simulink model "First_HIL_Scenario2"  (R2023a)
settings: Solver=ode1  StartTime=0.0  StopTime=inf  FixedStep=0.001  RelTol=1e-3
undefined symbols (not defined in the file or in its folder): ACC_X, ACC_Y, ACC_Z, Altitude, distance, GetTimeDemo, Gyro_X, Gyro_Y, Gyro_Z, Heading, Lane_Car_Distance_Left, Lane_Car_Distance_Right, Lane_Class, Lane_Coefficient_C0, Lane_Coefficient_C1, Lane_Coefficient_C2, Lane_Coefficient_C3, Lane_Curvature, Lane_Distance, Lane_ID, Latitude, Longitude, OBJ_Class, OBJ_Height, OBJ_ID, OBJ_Length, OBJ_RCS, OBJ_S_Azimuth, OBJ_S_Elevation, OBJ_S_Range, OBJ_S_Velocity, OBJ_Velocity, OBJ_Width, OBJ_X, OBJ_Y, OBJ_Z, Pitch, Roll, Subsystem, time, Timestamp, TrafficLight_Direction, TrafficLight_State, TrafficLight_Timer, Velocity, width, x, x1, x2, x3, x4, y, y1, y2, y3, y4, Yaw
(part 1 of 4)
Description:
  | 22222
settings Model: Creator=15751  LastModifiedBy=owner
settings SolverCC: AlgebraicLoopSolver=TrustRegion
settings OptimizationCC: LifeSpan=inf
settings DebuggingCC: MultiTaskRateTransMsg=warning  UnconnectedInputMsg=warning  UnconnectedOutputMsg=warning  UnconnectedLineMsg=warning  RootOutportRequireBusObject=error  StrictBusMsg=ErrorOnBusTreatedAsVector  ArithmeticOperatorsInVariantConditions=warning
settings HardwareCC: ProdBitPerPointer=32  ProdBitPerSizeT=32  ProdBitPerPtrDiffT=32  ProdLargestAtomicFloat=None  ProdWordSize=32  ProdHWDeviceType=Intel->x86/Pentium
settings ModelReferenceCC: EnableRefExpFcnMdlSchedulingChecks=on
settings SFSimCC: CustomCodeUndefinedFunction=UseInterfaceOnly
settings RTWCC: Description=NI Phar Lap Real-Time & Windows Targets  SystemTargetFile=NIVeriStand.tlc  TemplateMakefile=NIVeriStand_vc.tmf
settings RTWCC: CustomInclude=|
  | C:\Program Files\PanoSim5\Bin\SimulinkLib\dependence\NI
  | C:\Program
  | Files\PanoSim5\Bin\SimulinkLib\dependence\NI
settings RTWCC: CustomSource=|
  | DataReceiver.c
  | DataSender.c
  | udpFunc.c
settings CodeAppCC: StateflowObjectComments=on
settings STFCustomTargetCC: TargetLangStandard=C89/C90 (ANSI)  ConcurrentExecutionCompliant=off  MatFileLogging=on  MATLABClassNameForMDSCustomization=Simulink.SoftwareTarget.TargetSpecificTriggerConfigurationBase  UseToolchainInfoCompliant=off  SystemTargetFile=NIVeriStand.tlc
settings SimscapeCC: SimscapeNormalizeSystem=off

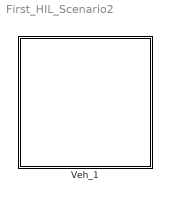
== system First_HIL_Scenario2 ==
  Veh_1 : Subsystem  Tag=PanoSim_System
      mask Display: image(imread('Sedan_2.jpg'));color('white');text(0,0,'Veh_1','HorizontalAlignment','left','verticalAlignment','bottom');color('red');text(0.1,0.1,'P','HorizontalAlignment','right','verticalAlignment','top');

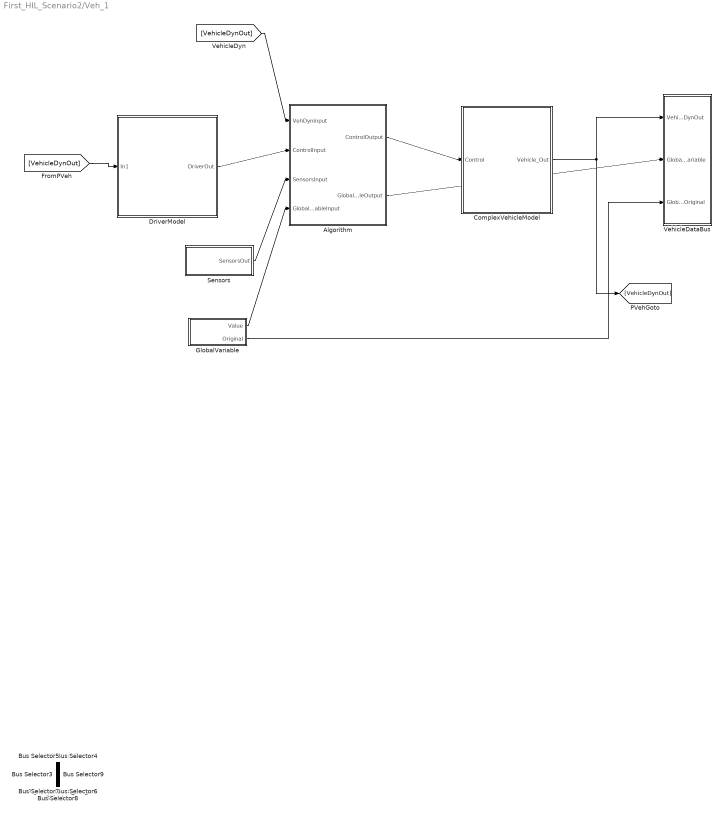
== system First_HIL_Scenario2/Veh_1 ==
  Algorithm : Subsystem
  Algorithm/Test_Bus_Selector : BusSelector  OutputSignals=signal1,signal2
  Bus Selector{1..9} (9 alike) : BusSelector  OutputSignals=signal1,signal2
  ComplexVehicleModel : Subsystem
  DriverModel : Subsystem  Tag=PanoSim_System
      mask Display: image(imread('driver.jpg'))
  GlobalVariable : Subsystem
  Sensors : Subsystem
  VehicleDataBus : Subsystem
  wires:
  Algorithm/2(GlobalVariableOutput) -> VehicleDataBus/2(GlobalVariable)
  Algorithm/1(ControlOutput) -> ComplexVehicleModel/1(Control)
  GlobalVariable/1(Value) -> Algorithm/4(GlobalVariableInput)
  Sensors/1(SensorsOut) -> Algorithm/3(SensorsInput)
  DriverModel/1(DriverOut) -> Algorithm/2(ControlInput)
  [VehicleDynOut] -> Algorithm/1(VehDynInput)
  GlobalVariable/2(Original) -> VehicleDataBus/3(GlobalVariableOriginal)
  [VehicleDynOut] -> DriverModel/1(In1)
  ComplexVehicleModel/1(Vehicle_Out) -> VehicleDataBus/1(VehicleDynOut), [VehicleDynOut]
